simulink model "PM_fnc100_DevHarness"  (R2022a)
settings: Solver=FixedStepDiscrete  StartTime=1  StopTime=inf  FixedStep=1  RelTol=1e-3
values from neighbouring files (symbols this model uses):
  fixedsteprate_s = rate_s    (= 0.01)    [PM_fnc1000_tc01_iter01_testsignal_builder.m]    (also in PM_fnc21_tc01_iter01_testsignal_builder.m; PM_fnc22_tc01_iter01_testsignal_builder.m)
undefined symbols (not defined in the file or in its folder): cal_abs_ampslimit_hyst_A, cal_abs_ampslimit_thresh_A, cal_chg_falling_slew_rate, cal_chg_PL1_ini, cal_chg_rising_slew_rate, cal_ChgPL1_expiry_dur_thresh_ms, cal_ChgPL1_restore_dur_thresh_ms, cal_ChgPL2_expiry_dur_thresh_ms, cal_ChgPL2_restore_dur_thresh_ms, cal_dchg_falling_slew_rate, cal_dchg_PL1_ini, cal_dchg_rising_slew_rate, cal_DchgPL1_expiry_dur_thresh_ms, cal_DchgPL1_restore_dur_thresh_ms, cal_DchgPL2_expiry_dur_thresh_ms, cal_DchgPL2_restore_dur_thresh_ms, cal_table_cell_soc_percent, cal_table_cell_temp_degC, cal_table_DchgPL1_10s_limits_xtempysoc, cal_table_DchgPL1_60s_limits_xtempysoc, cal_table_DchgPL1_cont_limits_xtempysoc, scaler
libraries: PM_lib x6
settings Model: PacingRate=1.600000  Creator=306427  LastModifiedBy=306427
settings SolverCC: ZeroCrossAlgorithm=Adaptive

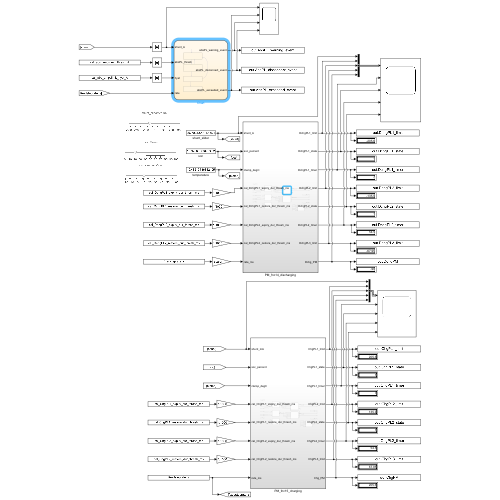
[thumbnail: Simulink's stored preview of the top-level diagram]
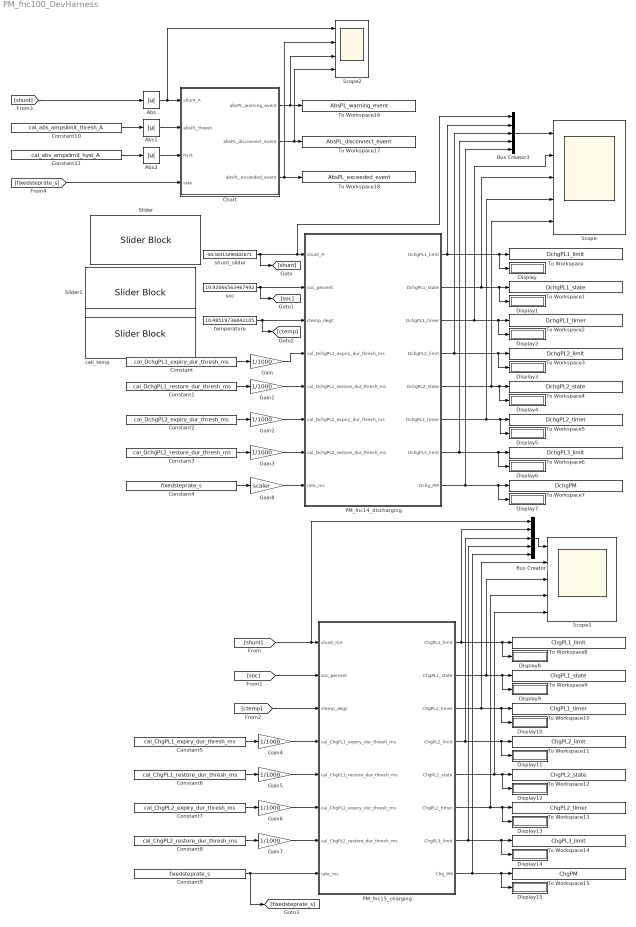
== system PM_fnc100_DevHarness ==
  Abs : Abs  SaturateOnIntegerOverflow=off
  Abs1 : Abs  SaturateOnIntegerOverflow=off
  Abs2 : Abs  SaturateOnIntegerOverflow=off
  Bus Creator1 : BusCreator  Inputs=5
  Bus Creator3 : BusCreator  Inputs=5
  Chart : Stateflow chart  TreatAsAtomicUnit=on
  Constant : Constant  Value=cal_DchgPL1_expiry_dur_thresh_ms
  Constant1 : Constant  Value=cal_DchgPL1_restore_dur_thresh_ms
  Constant10 : Constant  Value=cal_abs_ampslimit_thresh_A
  Constant11 : Constant  Value=cal_abs_ampslimit_hyst_A
  Constant2 : Constant  Value=cal_DchgPL2_expiry_dur_thresh_ms
  Constant3 : Constant  Value=cal_DchgPL2_restore_dur_thresh_ms
  Constant4 : Constant  Value=fixedsteprate_s
  Constant5 : Constant  Value=cal_ChgPL1_expiry_dur_thresh_ms
  Constant6 : Constant  Value=cal_ChgPL1_restore_dur_thresh_ms
  Constant7 : Constant  Value=cal_ChgPL2_expiry_dur_thresh_ms
  Constant8 : Constant  Value=cal_ChgPL2_restore_dur_thresh_ms
  Constant9 : Constant  Value=fixedsteprate_s
  Display{,1..15} (16 alike) : Display
  Gain{,1..7} (8 alike) : Gain  Gain=1/1000
  Gain8 : Gain  Gain=scaler
  PM_fnc14_discharging : Subsystem
  PM_fnc15_charging : Subsystem
  Scope : Scope  NumInputPorts=5
  Scope1 : Scope  NumInputPorts=5
  Scope2 : Scope  NumInputPorts=4
  Slider : SliderBlock  ScaleMin=-300  ScaleMax=300
  Slider1 : SliderBlock
  To Workspace : ToWorkspace  VariableName=DchgPL1_limit  SampleTime=-1
      settings: Save2DSignal=2-D array (concatenate along first dimension)
  To Workspace1 : ToWorkspace  VariableName=DchgPL1_state  SampleTime=-1
      settings: Save2DSignal=2-D array (concatenate along first dimension)
  To Workspace10 : ToWorkspace  VariableName=ChgPL1_timer  SampleTime=-1
      settings: Save2DSignal=2-D array (concatenate along first dimension)
  To Workspace11 : ToWorkspace  VariableName=ChgPL2_limit  SampleTime=-1
      settings: Save2DSignal=2-D array (concatenate along first dimension)
  To Workspace12 : ToWorkspace  VariableName=ChgPL2_state  SampleTime=-1
      settings: Save2DSignal=2-D array (concatenate along first dimension)
  To Workspace13 : ToWorkspace  VariableName=ChgPL2_timer  SampleTime=-1
      settings: Save2DSignal=2-D array (concatenate along first dimension)
  To Workspace14 : ToWorkspace  VariableName=ChgPL3_limit  SampleTime=-1
      settings: Save2DSignal=2-D array (concatenate along first dimension)
  To Workspace15 : ToWorkspace  VariableName=ChgPM  SampleTime=-1
      settings: Save2DSignal=2-D array (concatenate along first dimension)
  To Workspace16 : ToWorkspace  VariableName=AbsPL_warning_event  SampleTime=-1
      settings: Save2DSignal=2-D array (concatenate along first dimension)
  To Workspace17 : ToWorkspace  VariableName=AbsPL_disconnect_event  SampleTime=-1
      settings: Save2DSignal=2-D array (concatenate along first dimension)
  To Workspace18 : ToWorkspace  VariableName=AbsPL_exceeded_event  SampleTime=-1
      settings: Save2DSignal=2-D array (concatenate along first dimension)
  To Workspace2 : ToWorkspace  VariableName=DchgPL1_timer  SampleTime=-1
      settings: Save2DSignal=2-D array (concatenate along first dimension)
  To Workspace3 : ToWorkspace  VariableName=DchgPL2_limit  SampleTime=-1
      settings: Save2DSignal=2-D array (concatenate along first dimension)
  To Workspace4 : ToWorkspace  VariableName=DchgPL2_state  SampleTime=-1
      settings: Save2DSignal=2-D array (concatenate along first dimension)
  To Workspace5 : ToWorkspace  VariableName=DchgPL2_timer  SampleTime=-1
      settings: Save2DSignal=2-D array (concatenate along first dimension)
  To Workspace6 : ToWorkspace  VariableName=DchgPL3_limit  SampleTime=-1
      settings: Save2DSignal=2-D array (concatenate along first dimension)
  To Workspace7 : ToWorkspace  VariableName=DchgPM  SampleTime=-1
      settings: Save2DSignal=2-D array (concatenate along first dimension)
  To Workspace8 : ToWorkspace  VariableName=ChgPL1_limit  SampleTime=-1
      settings: Save2DSignal=2-D array (concatenate along first dimension)
  To Workspace9 : ToWorkspace  VariableName=ChgPL1_state  SampleTime=-1
      settings: Save2DSignal=2-D array (concatenate along first dimension)
  cell_temp : SliderBlock  ScaleMin=-20  ScaleMax=65
  shunt_slider : Constant  Value=-56.58313290402671
  soc : Constant  Value=19.92066563467492
  temperature : Constant  Value=10.48519736842105
  wires:
  soc/1 -> [soc], PM_fnc14_discharging/2(soc_percent)
  temperature/1 -> [ctemp], PM_fnc14_discharging/3(ctemp_degC)
  Constant/1 -> Gain/1
  Constant1/1 -> Gain1/1
  Constant2/1 -> Gain2/1
  Constant3/1 -> Gain3/1
  Constant4/1 -> Gain8/1
  shunt_slider/1 -> Bus Creator3/1, PM_fnc14_discharging/1(shunt_A), [shunt]
  PM_fnc14_discharging/1(DchgPL1_limit) -> Bus Creator3/2, Display/1, To Workspace/1
  PM_fnc14_discharging/2(DchgPL1_state) -> Display1/1, To Workspace1/1, Scope/3
  PM_fnc14_discharging/3(DchgPL1_timer) -> To Workspace2/1, Display2/1, Scope/2
  PM_fnc14_discharging/4(DchgPL2_limit) -> To Workspace3/1, Display3/1, Bus Creator3/3
  PM_fnc14_discharging/5(DchgPL2_state) -> Display4/1, To Workspace4/1, Scope/5
  PM_fnc14_discharging/7(DchgPL3_limit) -> Display6/1, To Workspace6/1, Bus Creator3/4
  Gain/1 -> PM_fnc14_discharging/4(cal_DchgPL1_expiry_dur_thresh_ms)
  Gain1/1 -> PM_fnc14_discharging/5(cal_DchgPL1_restore_dur_thresh_ms)
  Gain2/1 -> PM_fnc14_discharging/6(cal_DchgPL2_expiry_dur_thresh_ms)
  Gain3/1 -> PM_fnc14_discharging/7(cal_DchgPL2_restore_dur_thresh_ms)
  Bus Creator3/1 -> Scope/1
  PM_fnc14_discharging/6(DchgPL2_timer) -> Display5/1, To Workspace5/1, Scope/4
  PM_fnc14_discharging/8(Dchg_PM) -> Display7/1, To Workspace7/1, Bus Creator3/5
  Gain7/1 -> PM_fnc15_charging/7(cal_ChgPL2_restore_dur_thresh_ms)
  PM_fnc15_charging/6(ChgPL2_timer) -> To Workspace13/1, Display13/1, Scope1/4
  Constant8/1 -> Gain7/1
  Gain6/1 -> PM_fnc15_charging/6(cal_ChgPL2_expiry_dur_thresh_ms)
  Gain5/1 -> PM_fnc15_charging/5(cal_ChgPL1_restore_dur_thresh_ms)
  Gain4/1 -> PM_fnc15_charging/4(cal_ChgPL1_expiry_dur_thresh_ms)
  Constant5/1 -> Gain4/1
  Constant7/1 -> Gain6/1
  PM_fnc15_charging/7(ChgPL3_limit) -> To Workspace14/1, Display14/1, Bus Creator1/4
  PM_fnc15_charging/3(ChgPL1_timer) -> To Workspace10/1, Display10/1, Scope1/2
  PM_fnc15_charging/5(ChgPL2_state) -> To Workspace12/1, Display12/1, Scope1/5
  PM_fnc15_charging/8(Chg_PM) -> Bus Creator1/5, Display15/1, To Workspace15/1
  [shunt] -> Bus Creator1/1, PM_fnc15_charging/1(shunt_mA)
  [ctemp] -> PM_fnc15_charging/3(ctemp_degC)
  Constant6/1 -> Gain5/1
  Constant9/1 -> [fixedsteprate_s], PM_fnc15_charging/8(rate_ms)
  PM_fnc15_charging/4(ChgPL2_limit) -> To Workspace11/1, Display11/1, Bus Creator1/3
  [soc] -> PM_fnc15_charging/2(soc_percent)
  Bus Creator1/1 -> Scope1/1
  PM_fnc15_charging/2(ChgPL1_state) -> To Workspace9/1, Display9/1, Scope1/3
  PM_fnc15_charging/1(ChgPL1_limit) -> To Workspace8/1, Display8/1, Bus Creator1/2
  [shunt] -> Abs/1
  Constant10/1 -> Abs1/1
  Abs1/1 -> Chart/2(absPL_thresh)
  Abs/1 -> Scope2/1, Chart/1(shunt_A)
  Constant11/1 -> Abs2/1
  Abs2/1 -> Chart/3(hyst)
  [fixedsteprate_s] -> Chart/4(rate)
  Chart/1(absPL_warning_event) -> To Workspace16/1, Scope2/3
  Chart/2(absPL_disconnect_event) -> To Workspace17/1, Scope2/4
  Chart/3(absPL_exceeded_event) -> Scope2/2, To Workspace18/1
  Gain8/1 -> PM_fnc14_discharging/8(rate_ms)

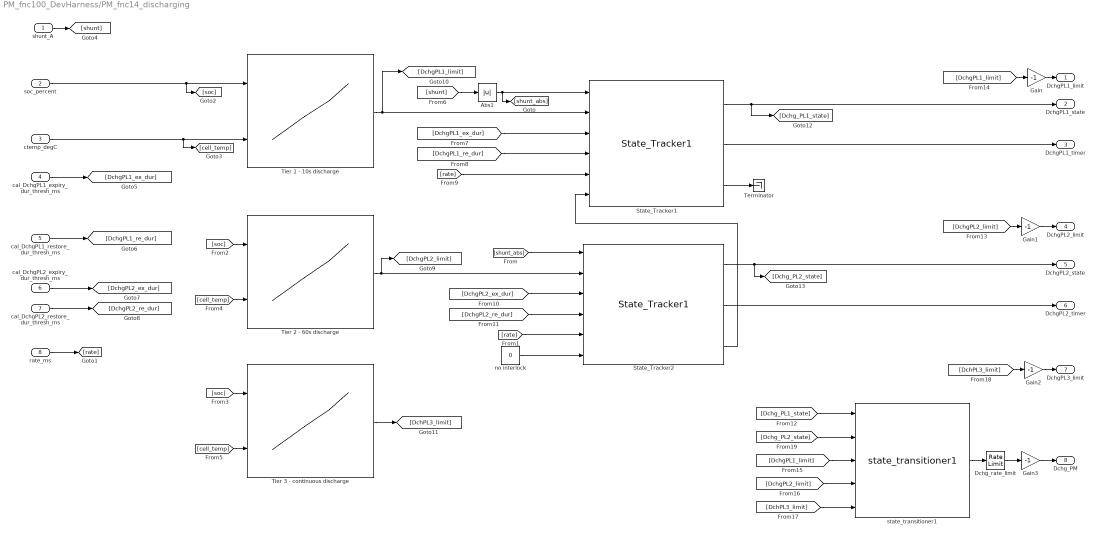
== system PM_fnc100_DevHarness/PM_fnc14_discharging ==
  shunt_A : Inport
  soc_percent : Inport  Port=2
  ctemp_degC : Inport  Port=3
  cal_DchgPL1_expiry_dur_thresh_ms : Inport  Port=4
  cal_DchgPL1_restore_dur_thresh_ms : Inport  Port=5
  cal_DchgPL2_expiry_dur_thresh_ms : Inport  Port=6
  cal_DchgPL2_restore_dur_thresh_ms : Inport  Port=7
  rate_ms : Inport  Port=8
  Abs1 : Abs  SaturateOnIntegerOverflow=off
  Dchg_rate_limit : RateLimiter  RisingSlewLimit=cal_dchg_rising_slew_rate  FallingSlewLimit=cal_dchg_falling_slew_rate  SampleTimeMode=inherited  InitialCondition=cal_dchg_PL1_ini
  Gain{,1..3} (4 alike) : Gain  Gain=-1
  State_Tracker1 : PM_lib/State_Tracker1  SystemSampleTime=-1  VariantActivationTime=update diagram  Latency=0  AutoFrameSizeCalculation=off
  State_Tracker2 : PM_lib/State_Tracker1  SystemSampleTime=-1  VariantActivationTime=update diagram  Latency=0  AutoFrameSizeCalculation=off
  Terminator : Terminator
  Tier 1 - 10s discharge : Lookup_n-D  BreakpointsForDimension1=cal_table_cell_soc_percent  BreakpointsForDimension2=cal_table_cell_temp_degC  Table=cal_table_DchgPL1_10s_limits_xtempysoc  InternalRulePriority=Speed  RndMeth=Simplest
      settings: InputPortMap=u0,u1
  Tier 2 - 60s discharge : Lookup_n-D  BreakpointsForDimension1=cal_table_cell_soc_percent  BreakpointsForDimension2=cal_table_cell_temp_degC  Table=cal_table_DchgPL1_60s_limits_xtempysoc  InternalRulePriority=Speed  RndMeth=Simplest
      settings: InputPortMap=u0,u1
  Tier 3 - continuous discharge : Lookup_n-D  BreakpointsForDimension1=cal_table_cell_soc_percent  BreakpointsForDimension2=cal_table_cell_temp_degC  Table=cal_table_DchgPL1_cont_limits_xtempysoc  InternalRulePriority=Speed  RndMeth=Simplest
      settings: InputPortMap=u0,u1
  no interlock : Constant  Value=0  OutDataTypeStr=boolean
  state_transitioner1 : PM_lib/state_transitioner1  SystemSampleTime=-1  VariantActivationTime=update diagram  Latency=0  AutoFrameSizeCalculation=off
  DchgPL1_limit : Outport
  DchgPL1_state : Outport  Port=2
  DchgPL1_timer : Outport  Port=3
  DchgPL2_limit : Outport  Port=4
  DchgPL2_state : Outport  Port=5
  DchgPL2_timer : Outport  Port=6
  DchgPL3_limit : Outport  Port=7
  Dchg_PM : Outport  Port=8
  wires:
  [cell_temp] -> Tier 3 - continuous discharge/2
  State_Tracker2/2 -> DchgPL2_timer/1
  [soc] -> Tier 2 - 60s discharge/1
  [cell_temp] -> Tier 2 - 60s discharge/2
  ctemp_degC/1 -> [cell_temp], Tier 1 - 10s discharge/2
  [rate] -> State_Tracker1/5
  cal_DchgPL2_expiry_dur_thresh_ms/1 -> [DchgPL2_ex_dur]
  Tier 2 - 60s discharge/1 -> [DchgPL2_limit], State_Tracker2/2
  State_Tracker2/1 -> [Dchg_PL2_state], DchgPL2_state/1
  State_Tracker1/2 -> DchgPL1_timer/1
  State_Tracker1/1 -> [Dchg_PL1_state], DchgPL1_state/1
  [rate] -> State_Tracker2/5
  [soc] -> Tier 3 - continuous discharge/1
  rate_ms/1 -> [rate]
  cal_DchgPL1_expiry_dur_thresh_ms/1 -> [DchgPL1_ex_dur]
  [shunt_abs] -> State_Tracker2/1
  Abs1/1 -> State_Tracker1/1, [shunt_abs]
  shunt_A/1 -> [shunt]
  cal_DchgPL1_restore_dur_thresh_ms/1 -> [DchgPL1_re_dur]
  Tier 1 - 10s discharge/1 -> [DchgPL1_limit], State_Tracker1/2
  soc_percent/1 -> [soc], Tier 1 - 10s discharge/1
  cal_DchgPL2_restore_dur_thresh_ms/1 -> [DchgPL2_re_dur]
  [shunt] -> Abs1/1
  [DchgPL2_re_dur] -> State_Tracker2/4
  [DchgPL2_ex_dur] -> State_Tracker2/3
  [DchgPL1_re_dur] -> State_Tracker1/4
  [DchgPL1_ex_dur] -> State_Tracker1/3
  no interlock/1 -> State_Tracker2/6
  State_Tracker2/3 -> State_Tracker1/6
  State_Tracker1/3 -> Terminator/1
  state_transitioner1/1 -> Dchg_rate_limit/1
  [DchgPL2_limit] -> Gain1/1
  [DchgPL1_limit] -> Gain/1
  [DchgPL1_limit] -> state_transitioner1/3
  [DchgPL2_limit] -> state_transitioner1/4
  Tier 3 - continuous discharge/1 -> [DchPL3_limit]
  [DchPL3_limit] -> state_transitioner1/5
  [DchPL3_limit] -> Gain2/1
  Gain/1 -> DchgPL1_limit/1
  Gain1/1 -> DchgPL2_limit/1
  Gain2/1 -> DchgPL3_limit/1
  Gain3/1 -> Dchg_PM/1
  [Dchg_PL1_state] -> state_transitioner1/1
  [Dchg_PL2_state] -> state_transitioner1/2
  Dchg_rate_limit/1 -> Gain3/1

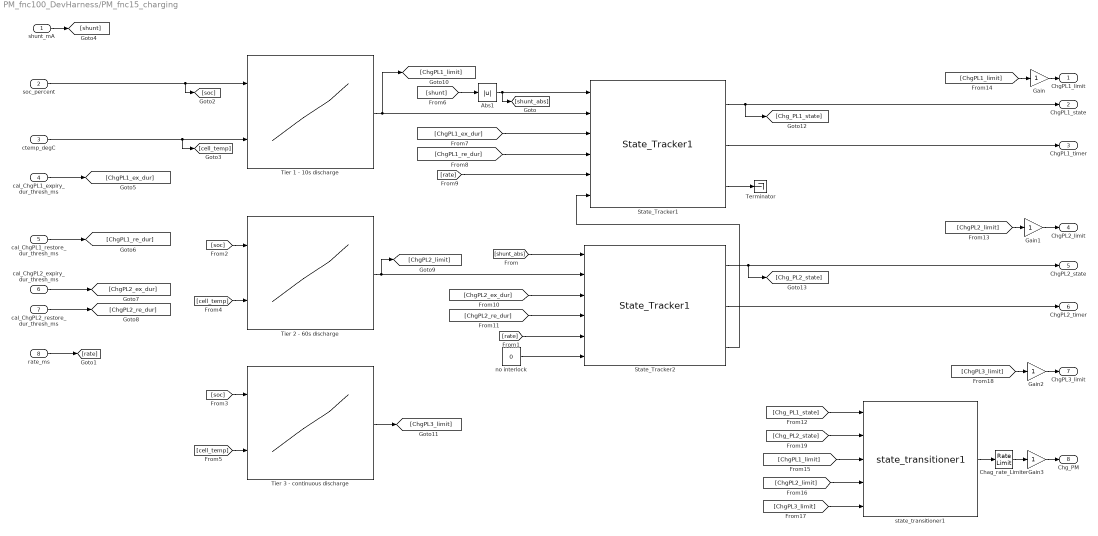
== system PM_fnc100_DevHarness/PM_fnc15_charging ==
  shunt_mA : Inport
  soc_percent : Inport  Port=2
  ctemp_degC : Inport  Port=3
  cal_ChgPL1_expiry_dur_thresh_ms : Inport  Port=4
  cal_ChgPL1_restore_dur_thresh_ms : Inport  Port=5
  cal_ChgPL2_expiry_dur_thresh_ms : Inport  Port=6
  cal_ChgPL2_restore_dur_thresh_ms : Inport  Port=7
  rate_ms : Inport  Port=8
  Abs1 : Abs  SaturateOnIntegerOverflow=off
  Chag_rate_Limiter : RateLimiter  RisingSlewLimit=cal_chg_rising_slew_rate  FallingSlewLimit=cal_chg_falling_slew_rate  SampleTimeMode=inherited  InitialCondition=cal_chg_PL1_ini
  Gain{,1..3} (4 alike) : Gain
  State_Tracker1 : PM_lib/State_Tracker1  SystemSampleTime=-1  VariantActivationTime=update diagram  Latency=0  AutoFrameSizeCalculation=off
  State_Tracker2 : PM_lib/State_Tracker1  SystemSampleTime=-1  VariantActivationTime=update diagram  Latency=0  AutoFrameSizeCalculation=off
  Terminator : Terminator
  Tier 1 - 10s discharge : Lookup_n-D  BreakpointsForDimension1=cal_table_cell_soc_percent  BreakpointsForDimension2=cal_table_cell_temp_degC  Table=cal_table_DchgPL1_10s_limits_xtempysoc  InternalRulePriority=Speed  RndMeth=Simplest
      settings: InputPortMap=u0,u1
  Tier 2 - 60s discharge : Lookup_n-D  BreakpointsForDimension1=cal_table_cell_soc_percent  BreakpointsForDimension2=cal_table_cell_temp_degC  Table=cal_table_DchgPL1_60s_limits_xtempysoc  InternalRulePriority=Speed  RndMeth=Simplest
      settings: InputPortMap=u0,u1
  Tier 3 - continuous discharge : Lookup_n-D  BreakpointsForDimension1=cal_table_cell_soc_percent  BreakpointsForDimension2=cal_table_cell_temp_degC  Table=cal_table_DchgPL1_cont_limits_xtempysoc  InternalRulePriority=Speed  RndMeth=Simplest
      settings: InputPortMap=u0,u1
  no interlock : Constant  Value=0  OutDataTypeStr=boolean
  state_transitioner1 : PM_lib/state_transitioner1  SystemSampleTime=-1  VariantActivationTime=update diagram  Latency=0  AutoFrameSizeCalculation=off
  ChgPL1_limit : Outport
  ChgPL1_state : Outport  Port=2
  ChgPL1_timer : Outport  Port=3
  ChgPL2_limit : Outport  Port=4
  ChgPL2_state : Outport  Port=5
  ChgPL2_timer : Outport  Port=6
  ChgPL3_limit : Outport  Port=7
  Chg_PM : Outport  Port=8
  wires:
  [cell_temp] -> Tier 3 - continuous discharge/2
  State_Tracker2/2 -> ChgPL2_timer/1
  [soc] -> Tier 2 - 60s discharge/1
  [cell_temp] -> Tier 2 - 60s discharge/2
  ctemp_degC/1 -> [cell_temp], Tier 1 - 10s discharge/2
  [rate] -> State_Tracker1/5
  cal_ChgPL2_expiry_dur_thresh_ms/1 -> [ChgPL2_ex_dur]
  Tier 2 - 60s discharge/1 -> [ChgPL2_limit], State_Tracker2/2
  State_Tracker2/1 -> [Chg_PL2_state], ChgPL2_state/1
  State_Tracker1/2 -> ChgPL1_timer/1
  State_Tracker1/1 -> [Chg_PL1_state], ChgPL1_state/1
  [rate] -> State_Tracker2/5
  [soc] -> Tier 3 - continuous discharge/1
  rate_ms/1 -> [rate]
  cal_ChgPL1_expiry_dur_thresh_ms/1 -> [ChgPL1_ex_dur]
  [shunt_abs] -> State_Tracker2/1
  Abs1/1 -> State_Tracker1/1, [shunt_abs]
  shunt_mA/1 -> [shunt]
  cal_ChgPL1_restore_dur_thresh_ms/1 -> [ChgPL1_re_dur]
  Tier 1 - 10s discharge/1 -> [ChgPL1_limit], State_Tracker1/2
  soc_percent/1 -> [soc], Tier 1 - 10s discharge/1
  cal_ChgPL2_restore_dur_thresh_ms/1 -> [ChgPL2_re_dur]
  [shunt] -> Abs1/1
  [ChgPL2_re_dur] -> State_Tracker2/4
  [ChgPL2_ex_dur] -> State_Tracker2/3
  [ChgPL1_re_dur] -> State_Tracker1/4
  [ChgPL1_ex_dur] -> State_Tracker1/3
  no interlock/1 -> State_Tracker2/6
  State_Tracker2/3 -> State_Tracker1/6
  State_Tracker1/3 -> Terminator/1
  state_transitioner1/1 -> Chag_rate_Limiter/1
  [ChgPL2_limit] -> Gain1/1
  [ChgPL1_limit] -> Gain/1
  [ChgPL1_limit] -> state_transitioner1/3
  [ChgPL2_limit] -> state_transitioner1/4
  Tier 3 - continuous discharge/1 -> [ChgPL3_limit]
  [ChgPL3_limit] -> state_transitioner1/5
  [ChgPL3_limit] -> Gain2/1
  Gain/1 -> ChgPL1_limit/1
  Gain1/1 -> ChgPL2_limit/1
  Gain2/1 -> ChgPL3_limit/1
  Gain3/1 -> Chg_PM/1
  Chag_rate_Limiter/1 -> Gain3/1
  [Chg_PL1_state] -> state_transitioner1/1
  [Chg_PL2_state] -> state_transitioner1/2

== stateflow chart PM_fnc100_DevHarness/Chart ==
  state RESET
    timer = 0;
    absPL_exceeded_event = boolean(0);
    absPL_warning_event = boolean(0);
    absPL_disconnect_event = boolean(0);
  state MEAS_DURATION
    timer = timer + rate;
    absPL_exceeded_event = boolean(1);
    absPL_warning_event = boolean(0);
    absPL_disconnect_event = boolean(0);
  state WARNING
    timer = timer + rate;
    absPL_warning_event = boolean(1);
    absPL_disconnect_event = boolean(0);
  state DISCONNECT
    timer = timer + rate;
    absPL_disconnect_event = boolean(1);
  (default) -> RESET
  WARNING -> RESET [order 1] : [shunt_A < absPL_thresh - hyst]
  RESET -> MEAS_DURATION : [shunt_A > absPL_thresh]
  MEAS_DURATION -> RESET [order 2] : [shunt_A < absPL_thresh -hyst]
  MEAS_DURATION -> WARNING [order 1] : [timer >= 1]
  WARNING -> DISCONNECT [order 2] : [timer > 3]
  data: timer local; absPL_warning_event output; absPL_disconnect_event output; shunt_A input; absPL_thresh input; hyst input; rate input; absPL_exceeded_event output
